simulink model "test_kalman_scaling"  (R2024a)
settings: Solver=FixedStepAuto  StartTime=0.0  StopTime=4e-4  FixedStep=8e-9  RelTol=1e-3
values from neighbouring files (symbols this model uses):
  A1 = [0,                  1,  0, 0,   0, 0 ... (first row only)    [three_axis_plant_ver_0_init.m]
  A2 = [0,                  1,  0, 0,   0, 0 ... (first row only)    [three_axis_plant_ver_0_init.m]
  B1 = [0; p.C_f/p.m; 0; p.C_f_xz/p.m; 0; p.C_f_xy/p.m;]    [three_axis_plant_ver_0_init.m]
  C1 = [p.C_el_x,  0,         p.C_el_xz,    0, p.C_el_xy, 0;       0,         p.C_el_x,          0,    0,         0, 0;       p.C_el_zx,        0,   p.C_el_z,    0,    p.C_el_zy, 0]    [three_axis_plant_ver_0_init.m]
  eff_fun = @(V) cos(eff_w.*V.^2)./(eff_m*V.^4 + eff_n) + eff_p    [three_axis_plant_ver_0_init.m]
  G1 = [0 0 0; 1/p.m 0 0; 0 0 0; 0 1/p.m 0; 0 0 0; 0 0 1/p.m]    [three_axis_plant_ver_0_init.m]
  t_off = 2*T_max +(t_on + 100*(2*pi/abs(p.Omega_ip)))    [three_axis_plant_ver_0_init.m]
  t_on = 0*2*T_max*0.01    [three_axis_plant_ver_0_init.m]
undefined symbols (not defined in the file or in its folder): clqr, k, lqg, p, xc7z020clg400
libraries: hdlSSR x61, hdlBasic x40, simulink x10, vmcUtilities x1
(part 2 of 2)

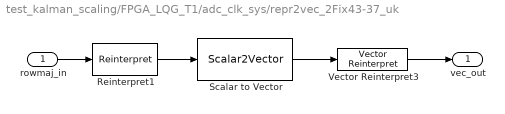
== system test_kalman_scaling/FPGA_LQG_T1/adc_clk_sys/repr2vec_2Fix43-37_uk ==
  rowmaj_in : Inport
  Reinterpret1 : hdlBasic/Reinterpret  force_arith_type=on  arith_type=Unsigned  force_bin_pt=on  bin_pt=0  XmcBlockStatus=1  maskContainerNames=group1  block_type=reinterpret  block_config=sysgen:Reinterpret_config
  Scalar to Vector : hdlSSR/Scalar2Vector  Width=43  sg_ssr=2  block_type=scalar2vector_ssr  XmcBlockStatus=1  sg_ssr_prev=2  maskContainerNames=group1
  Vector Reinterpret3 : hdlSSR/Vector Reinterpret  force_arith_type=on  arith_type="Signed  (2's comp)"  force_bin_pt=on  bin_pt=37  sg_ssr=2  block_type=reinterpret_ssr  XmcBlockStatus=1  sg_ssr_prev=2  maskContainerNames=group1
  vec_out : Outport
  wires:
  Scalar to Vector/1 -> Vector Reinterpret3/1
  Reinterpret1/1 -> Scalar to Vector/1
  rowmaj_in/1 -> Reinterpret1/1
  Vector Reinterpret3/1 -> vec_out/1

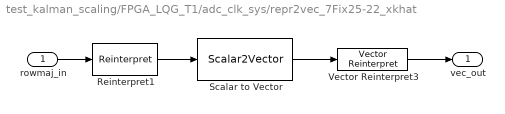
== system test_kalman_scaling/FPGA_LQG_T1/adc_clk_sys/repr2vec_7Fix25-22_xkhat ==
  rowmaj_in : Inport
  Reinterpret1 : hdlBasic/Reinterpret  force_arith_type=on  arith_type=Unsigned  force_bin_pt=on  bin_pt=0  XmcBlockStatus=1  maskContainerNames=group1  block_type=reinterpret  block_config=sysgen:Reinterpret_config
  Scalar to Vector : hdlSSR/Scalar2Vector  Width=25  sg_ssr=7  block_type=scalar2vector_ssr  XmcBlockStatus=1  sg_ssr_prev=7  maskContainerNames=group1
  Vector Reinterpret3 : hdlSSR/Vector Reinterpret  force_arith_type=on  arith_type="Signed  (2's comp)"  force_bin_pt=on  bin_pt=22  sg_ssr=7  block_type=reinterpret_ssr  XmcBlockStatus=1  sg_ssr_prev=7  maskContainerNames=group1
  vec_out : Outport
  wires:
  Scalar to Vector/1 -> Vector Reinterpret3/1
  Reinterpret1/1 -> Scalar to Vector/1
  rowmaj_in/1 -> Reinterpret1/1
  Vector Reinterpret3/1 -> vec_out/1

== system test_kalman_scaling/FPGA_LQG_T1/adc_clk_sys/vec2repr_14_Gamma_res ==
  vec_in : Inport
  Reinterpret2 : hdlBasic/Reinterpret  force_arith_type=on  arith_type=Unsigned  force_bin_pt=on  bin_pt=0  XmcBlockStatus=1  maskContainerNames=group1  block_type=reinterpret  block_config=sysgen:Reinterpret_config
  Vector Reinterpret2 : hdlSSR/Vector Reinterpret  force_arith_type=on  arith_type=Unsigned  force_bin_pt=on  bin_pt=0  sg_ssr=14  block_type=reinterpret_ssr  XmcBlockStatus=1  sg_ssr_prev=14  maskContainerNames=group1
  Vector to Scalar : hdlSSR/Vector2Scalar  sg_ssr=14  block_type=vector2scalar_ssr  XmcBlockStatus=1  sg_ssr_prev=14  maskContainerNames=group1
  rowmaj_out : Outport
  wires:
  Vector to Scalar/1 -> Reinterpret2/1
  Vector Reinterpret2/1 -> Vector to Scalar/1
  vec_in/1 -> Vector Reinterpret2/1
  Reinterpret2/1 -> rowmaj_out/1

== system test_kalman_scaling/FPGA_LQG_T1/adc_clk_sys/vec2repr_14_Gamma_shift ==
  vec_in : Inport
  Reinterpret2 : hdlBasic/Reinterpret  force_arith_type=on  arith_type=Unsigned  force_bin_pt=on  bin_pt=0  XmcBlockStatus=1  maskContainerNames=group1  block_type=reinterpret  block_config=sysgen:Reinterpret_config
  Vector Reinterpret2 : hdlSSR/Vector Reinterpret  force_arith_type=on  arith_type=Unsigned  force_bin_pt=on  bin_pt=0  sg_ssr=14  block_type=reinterpret_ssr  XmcBlockStatus=1  sg_ssr_prev=14  maskContainerNames=group1
  Vector to Scalar : hdlSSR/Vector2Scalar  sg_ssr=14  block_type=vector2scalar_ssr  XmcBlockStatus=1  sg_ssr_prev=14  maskContainerNames=group1
  rowmaj_out : Outport
  wires:
  Vector to Scalar/1 -> Reinterpret2/1
  Vector Reinterpret2/1 -> Vector to Scalar/1
  vec_in/1 -> Vector Reinterpret2/1
  Reinterpret2/1 -> rowmaj_out/1

== system test_kalman_scaling/FPGA_LQG_T1/adc_clk_sys/vec2repr_14_K_res ==
  vec_in : Inport
  Reinterpret2 : hdlBasic/Reinterpret  force_arith_type=on  arith_type=Unsigned  force_bin_pt=on  bin_pt=0  XmcBlockStatus=1  maskContainerNames=group1  block_type=reinterpret  block_config=sysgen:Reinterpret_config
  Vector Reinterpret2 : hdlSSR/Vector Reinterpret  force_arith_type=on  arith_type=Unsigned  force_bin_pt=on  bin_pt=0  sg_ssr=14  block_type=reinterpret_ssr  XmcBlockStatus=1  sg_ssr_prev=14  maskContainerNames=group1
  Vector to Scalar : hdlSSR/Vector2Scalar  sg_ssr=14  block_type=vector2scalar_ssr  XmcBlockStatus=1  sg_ssr_prev=14  maskContainerNames=group1
  rowmaj_out : Outport
  wires:
  Vector to Scalar/1 -> Reinterpret2/1
  Vector Reinterpret2/1 -> Vector to Scalar/1
  vec_in/1 -> Vector Reinterpret2/1
  Reinterpret2/1 -> rowmaj_out/1

== system test_kalman_scaling/FPGA_LQG_T1/adc_clk_sys/vec2repr_14_K_shift ==
  vec_in : Inport
  Reinterpret2 : hdlBasic/Reinterpret  force_arith_type=on  arith_type=Unsigned  force_bin_pt=on  bin_pt=0  XmcBlockStatus=1  maskContainerNames=group1  block_type=reinterpret  block_config=sysgen:Reinterpret_config
  Vector Reinterpret2 : hdlSSR/Vector Reinterpret  force_arith_type=on  arith_type=Unsigned  force_bin_pt=on  bin_pt=0  sg_ssr=14  block_type=reinterpret_ssr  XmcBlockStatus=1  sg_ssr_prev=14  maskContainerNames=group1
  Vector to Scalar : hdlSSR/Vector2Scalar  sg_ssr=14  block_type=vector2scalar_ssr  XmcBlockStatus=1  sg_ssr_prev=14  maskContainerNames=group1
  rowmaj_out : Outport
  wires:
  Vector to Scalar/1 -> Reinterpret2/1
  Vector Reinterpret2/1 -> Vector to Scalar/1
  vec_in/1 -> Vector Reinterpret2/1
  Reinterpret2/1 -> rowmaj_out/1

== system test_kalman_scaling/FPGA_LQG_T1/adc_clk_sys/vec2repr_14_L_res ==
  vec_in : Inport
  Reinterpret2 : hdlBasic/Reinterpret  force_arith_type=on  arith_type=Unsigned  force_bin_pt=on  bin_pt=0  XmcBlockStatus=1  maskContainerNames=group1  block_type=reinterpret  block_config=sysgen:Reinterpret_config
  Vector Reinterpret2 : hdlSSR/Vector Reinterpret  force_arith_type=on  arith_type=Unsigned  force_bin_pt=on  bin_pt=0  sg_ssr=14  block_type=reinterpret_ssr  XmcBlockStatus=1  sg_ssr_prev=14  maskContainerNames=group1
  Vector to Scalar : hdlSSR/Vector2Scalar  sg_ssr=14  block_type=vector2scalar_ssr  XmcBlockStatus=1  sg_ssr_prev=14  maskContainerNames=group1
  rowmaj_out : Outport
  wires:
  Vector to Scalar/1 -> Reinterpret2/1
  Vector Reinterpret2/1 -> Vector to Scalar/1
  vec_in/1 -> Vector Reinterpret2/1
  Reinterpret2/1 -> rowmaj_out/1

== system test_kalman_scaling/FPGA_LQG_T1/adc_clk_sys/vec2repr_14_L_shift ==
  vec_in : Inport
  Reinterpret2 : hdlBasic/Reinterpret  force_arith_type=on  arith_type=Unsigned  force_bin_pt=on  bin_pt=0  XmcBlockStatus=1  maskContainerNames=group1  block_type=reinterpret  block_config=sysgen:Reinterpret_config
  Vector Reinterpret2 : hdlSSR/Vector Reinterpret  force_arith_type=on  arith_type=Unsigned  force_bin_pt=on  bin_pt=0  sg_ssr=14  block_type=reinterpret_ssr  XmcBlockStatus=1  sg_ssr_prev=14  maskContainerNames=group1
  Vector to Scalar : hdlSSR/Vector2Scalar  sg_ssr=14  block_type=vector2scalar_ssr  XmcBlockStatus=1  sg_ssr_prev=14  maskContainerNames=group1
  rowmaj_out : Outport
  wires:
  Vector to Scalar/1 -> Reinterpret2/1
  Vector Reinterpret2/1 -> Vector to Scalar/1
  vec_in/1 -> Vector Reinterpret2/1
  Reinterpret2/1 -> rowmaj_out/1

== system test_kalman_scaling/FPGA_LQG_T1/adc_clk_sys/vec2repr_2 ==
  vec_in : Inport
  Reinterpret2 : hdlBasic/Reinterpret  force_arith_type=on  arith_type=Unsigned  force_bin_pt=on  bin_pt=0  XmcBlockStatus=1  maskContainerNames=group1  block_type=reinterpret  block_config=sysgen:Reinterpret_config
  Vector Reinterpret2 : hdlSSR/Vector Reinterpret  force_arith_type=on  arith_type=Unsigned  force_bin_pt=on  bin_pt=0  sg_ssr=2  block_type=reinterpret_ssr  XmcBlockStatus=1  sg_ssr_prev=2  maskContainerNames=group1
  Vector to Scalar : hdlSSR/Vector2Scalar  sg_ssr=2  block_type=vector2scalar_ssr  XmcBlockStatus=1  sg_ssr_prev=2  maskContainerNames=group1
  rowmaj_out : Outport
  wires:
  Vector to Scalar/1 -> Reinterpret2/1
  Vector Reinterpret2/1 -> Vector to Scalar/1
  vec_in/1 -> Vector Reinterpret2/1
  Reinterpret2/1 -> rowmaj_out/1

== system test_kalman_scaling/FPGA_LQG_T1/adc_clk_sys/vec2repr_2_uk ==
  vec_in : Inport
  Reinterpret2 : hdlBasic/Reinterpret  force_arith_type=on  arith_type=Unsigned  force_bin_pt=on  bin_pt=0  XmcBlockStatus=1  maskContainerNames=group1  block_type=reinterpret  block_config=sysgen:Reinterpret_config
  Vector Reinterpret2 : hdlSSR/Vector Reinterpret  force_arith_type=on  arith_type=Unsigned  force_bin_pt=on  bin_pt=0  sg_ssr=2  block_type=reinterpret_ssr  XmcBlockStatus=1  sg_ssr_prev=2  maskContainerNames=group1
  Vector to Scalar : hdlSSR/Vector2Scalar  sg_ssr=2  block_type=vector2scalar_ssr  XmcBlockStatus=1  sg_ssr_prev=2  maskContainerNames=group1
  rowmaj_out : Outport
  wires:
  Vector to Scalar/1 -> Reinterpret2/1
  Vector Reinterpret2/1 -> Vector to Scalar/1
  vec_in/1 -> Vector Reinterpret2/1
  Reinterpret2/1 -> rowmaj_out/1

== system test_kalman_scaling/FPGA_LQG_T1/adc_clk_sys/vec2repr_49_F_res ==
  vec_in : Inport
  Reinterpret2 : hdlBasic/Reinterpret  force_arith_type=on  arith_type=Unsigned  force_bin_pt=on  bin_pt=0  XmcBlockStatus=1  maskContainerNames=group1  block_type=reinterpret  block_config=sysgen:Reinterpret_config
  Vector Reinterpret2 : hdlSSR/Vector Reinterpret  force_arith_type=on  arith_type=Unsigned  force_bin_pt=on  bin_pt=0  sg_ssr=49  block_type=reinterpret_ssr  XmcBlockStatus=1  sg_ssr_prev=49  maskContainerNames=group1
  Vector to Scalar : hdlSSR/Vector2Scalar  sg_ssr=49  block_type=vector2scalar_ssr  XmcBlockStatus=1  sg_ssr_prev=49  maskContainerNames=group1
  rowmaj_out : Outport
  wires:
  Vector to Scalar/1 -> Reinterpret2/1
  Vector Reinterpret2/1 -> Vector to Scalar/1
  vec_in/1 -> Vector Reinterpret2/1
  Reinterpret2/1 -> rowmaj_out/1

== system test_kalman_scaling/FPGA_LQG_T1/adc_clk_sys/vec2repr_49_F_shift ==
  vec_in : Inport
  Reinterpret2 : hdlBasic/Reinterpret  force_arith_type=on  arith_type=Unsigned  force_bin_pt=on  bin_pt=0  XmcBlockStatus=1  maskContainerNames=group1  block_type=reinterpret  block_config=sysgen:Reinterpret_config
  Vector Reinterpret2 : hdlSSR/Vector Reinterpret  force_arith_type=on  arith_type=Unsigned  force_bin_pt=on  bin_pt=0  sg_ssr=49  block_type=reinterpret_ssr  XmcBlockStatus=1  sg_ssr_prev=49  maskContainerNames=group1
  Vector to Scalar : hdlSSR/Vector2Scalar  sg_ssr=49  block_type=vector2scalar_ssr  XmcBlockStatus=1  sg_ssr_prev=49  maskContainerNames=group1
  rowmaj_out : Outport
  wires:
  Vector to Scalar/1 -> Reinterpret2/1
  Vector Reinterpret2/1 -> Vector to Scalar/1
  vec_in/1 -> Vector Reinterpret2/1
  Reinterpret2/1 -> rowmaj_out/1

== system test_kalman_scaling/FPGA_LQG_T1/adc_clk_sys/accumulate_matmuls/repr2vec_7Fix43-37_B ==
  rowmaj_in : Inport
  Reinterpret1 : hdlBasic/Reinterpret  force_arith_type=on  arith_type=Unsigned  force_bin_pt=on  bin_pt=0  XmcBlockStatus=1  maskContainerNames=group1  block_type=reinterpret  block_config=sysgen:Reinterpret_config
  Scalar to Vector : hdlSSR/Scalar2Vector  Width=43  sg_ssr=7  block_type=scalar2vector_ssr  XmcBlockStatus=1  sg_ssr_prev=7  maskContainerNames=group1
  Vector Reinterpret3 : hdlSSR/Vector Reinterpret  force_arith_type=on  arith_type="Signed  (2's comp)"  force_bin_pt=on  bin_pt=37  sg_ssr=7  block_type=reinterpret_ssr  XmcBlockStatus=1  sg_ssr_prev=7  maskContainerNames=group1
  vec_out : Outport
  wires:
  Scalar to Vector/1 -> Vector Reinterpret3/1
  Reinterpret1/1 -> Scalar to Vector/1
  rowmaj_in/1 -> Reinterpret1/1
  Vector Reinterpret3/1 -> vec_out/1

== system test_kalman_scaling/FPGA_LQG_T1/adc_clk_sys/accumulate_matmuls/repr2vec_7Fix43-37_F ==
  rowmaj_in : Inport
  Reinterpret1 : hdlBasic/Reinterpret  force_arith_type=on  arith_type=Unsigned  force_bin_pt=on  bin_pt=0  XmcBlockStatus=1  maskContainerNames=group1  block_type=reinterpret  block_config=sysgen:Reinterpret_config
  Scalar to Vector : hdlSSR/Scalar2Vector  Width=43  sg_ssr=7  block_type=scalar2vector_ssr  XmcBlockStatus=1  sg_ssr_prev=7  maskContainerNames=group1
  Vector Reinterpret3 : hdlSSR/Vector Reinterpret  force_arith_type=on  arith_type="Signed  (2's comp)"  force_bin_pt=on  bin_pt=37  sg_ssr=7  block_type=reinterpret_ssr  XmcBlockStatus=1  sg_ssr_prev=7  maskContainerNames=group1
  vec_out : Outport
  wires:
  Scalar to Vector/1 -> Vector Reinterpret3/1
  Reinterpret1/1 -> Scalar to Vector/1
  rowmaj_in/1 -> Reinterpret1/1
  Vector Reinterpret3/1 -> vec_out/1

== system test_kalman_scaling/FPGA_LQG_T1/adc_clk_sys/accumulate_matmuls/repr2vec_7Fix43-37_L ==
  rowmaj_in : Inport
  Reinterpret1 : hdlBasic/Reinterpret  force_arith_type=on  arith_type=Unsigned  force_bin_pt=on  bin_pt=0  XmcBlockStatus=1  maskContainerNames=group1  block_type=reinterpret  block_config=sysgen:Reinterpret_config
  Scalar to Vector : hdlSSR/Scalar2Vector  Width=43  sg_ssr=7  block_type=scalar2vector_ssr  XmcBlockStatus=1  sg_ssr_prev=7  maskContainerNames=group1
  Vector Reinterpret3 : hdlSSR/Vector Reinterpret  force_arith_type=on  arith_type="Signed  (2's comp)"  force_bin_pt=on  bin_pt=37  sg_ssr=7  block_type=reinterpret_ssr  XmcBlockStatus=1  sg_ssr_prev=7  maskContainerNames=group1
  vec_out : Outport
  wires:
  Scalar to Vector/1 -> Vector Reinterpret3/1
  Reinterpret1/1 -> Scalar to Vector/1
  rowmaj_in/1 -> Reinterpret1/1
  Vector Reinterpret3/1 -> vec_out/1

== system test_kalman_scaling/FPGA_LQG_T1/adc_clk_sys/accumulate_matmuls/vec2repr_7 ==
  vec_in : Inport
  Reinterpret2 : hdlBasic/Reinterpret  force_arith_type=on  arith_type=Unsigned  force_bin_pt=on  bin_pt=0  XmcBlockStatus=1  maskContainerNames=group1  block_type=reinterpret  block_config=sysgen:Reinterpret_config
  Vector Reinterpret2 : hdlSSR/Vector Reinterpret  force_arith_type=on  arith_type=Unsigned  force_bin_pt=on  bin_pt=0  sg_ssr=7  block_type=reinterpret_ssr  XmcBlockStatus=1  sg_ssr_prev=7  maskContainerNames=group1
  Vector to Scalar : hdlSSR/Vector2Scalar  sg_ssr=7  block_type=vector2scalar_ssr  XmcBlockStatus=1  sg_ssr_prev=7  maskContainerNames=group1
  rowmaj_out : Outport
  wires:
  Vector to Scalar/1 -> Reinterpret2/1
  Vector Reinterpret2/1 -> Vector to Scalar/1
  vec_in/1 -> Vector Reinterpret2/1
  Reinterpret2/1 -> rowmaj_out/1

== matlab function test_kalman_scaling/Plant-Model (Reference)/MATLAB Function1 ==
  data: AP input; IP input; y output; sw input
function y = fcn(AP, IP, sw)

y = AP*abs(2-sw) + IP*abs(sw-1);

== matlab function test_kalman_scaling/Plant-Model (Reference)/MATLAB Function ==
  data: x input; F output; alpha input; beta input; delta input; dx_1 input; dx_0 input
function F = fcn(x, alpha, beta, delta, dx_1, dx_0)


F = (8*beta*exp(-(2*(dx_1 - x)^2)/delta^2)*(dx_1 - x))/delta^2 - (4*alpha*exp(-(2*(dx_0 - x)^2)/delta^2)*(dx_0 - x))/delta^2 - (16*beta*exp(-(2*(dx_1 - x)^2)/delta^2)*(dx_1 - x)^3)/delta^4;

== matlab function test_kalman_scaling/Plant-Model (Test 1)/MATLAB Function ==
  data: x input; F output; alpha input; beta input; delta input; dx_1 input; dx_0 input
function F = fcn(x, alpha, beta, delta, dx_1, dx_0)


F = (8*beta*exp(-(2*(dx_1 - x)^2)/delta^2)*(dx_1 - x))/delta^2 - (4*alpha*exp(-(2*(dx_0 - x)^2)/delta^2)*(dx_0 - x))/delta^2 - (16*beta*exp(-(2*(dx_1 - x)^2)/delta^2)*(dx_1 - x)^3)/delta^4;

== matlab function test_kalman_scaling/Plant-Model (Test 1)/MATLAB Function1 ==
  data: AP input; IP input; y output; sw input
function y = fcn(AP, IP, sw)

y = AP*abs(2-sw) + IP*abs(sw-1);
